simulink model "task1"  (R2024a)
settings: Solver=VariableStepAuto  StartTime=0.0  StopTime=10.0  RelTol=1e-8
values from neighbouring files (symbols this model uses):
  A = [8, 1, 11; 4, 0, 4; -4, -3, -7]    [main.m]
  B = [-1; -3; 3]    [main.m]
  K = K4    [main.m]
settings Model: Creator=alexivanov  LastModifiedBy=alexivanov

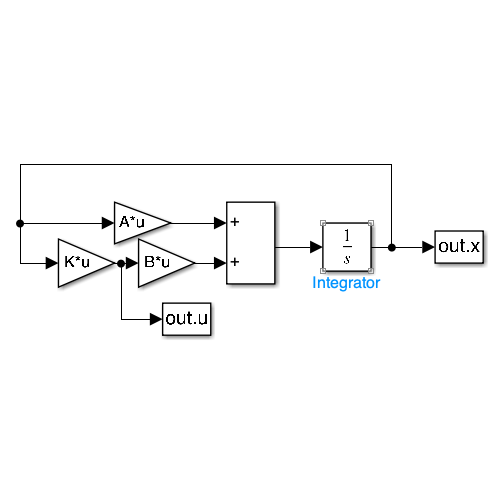
[thumbnail: Simulink's stored preview of the top-level diagram]
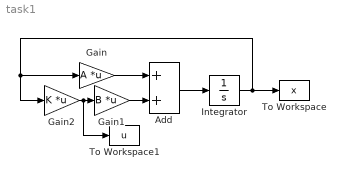
== system task1 ==
  Add : Sum
  Gain : Gain  Gain=A  Multiplication=Matrix(K*u)
  Gain1 : Gain  Gain=B  Multiplication=Matrix(K*u)
  Gain2 : Gain  Gain=K  Multiplication=Matrix(K*u)
  Integrator : Integrator  InitialCondition=[1; 1; 1]
  To Workspace : ToWorkspace  VariableName=x  SampleTime=-1
  To Workspace1 : ToWorkspace  VariableName=u  SampleTime=-1
  wires:
  Gain/1 -> Add/1
  Gain1/1 -> Add/2
  Gain2/1 -> To Workspace1/1, Gain1/1
  Integrator/1 -> To Workspace/1, Gain2/1, Gain/1
  Add/1 -> Integrator/1
